simulink model "MeUn_DD"  (R2016b)
settings: configuration reference "CodeGenConfigSet" (kept outside this file)
values from neighbouring files (symbols this model uses):
  DTY_CYC_MIN = fi(0,DutyCycle_rate)    [init_MeUn_DD.m]
  ErrorStatus = fi(0,State_uint8)    [init_MeUn_DD.m]
  MeUn_CrntCtlDT1Kd_C = Calibration.Parameter    [init_MeUn_DD.m]
  MeUn_CrntCtlDT1T1_C = Calibration.Parameter    [init_MeUn_DD.m]
  MeUn_nDiffMax_C = Calibration.Parameter    [init_MeUn_DD.m]
  MeUn_resCoil_C = Calibration.Parameter    [init_MeUn_DD.m]
  MeUn_rPwmOutMax_CUR = Calibration.Parameter    [init_MeUn_DD.m]
  MeUn_rPwmOutMax_CURX = Calibration.Parameter    [init_MeUn_DD.m]
  MeUn_rPwmOutMin_C = Calibration.Parameter    [init_MeUn_DD.m]
  MeUn_rSetLin_CUR = Calibration.Parameter    [init_MeUn_DD.m]
  MeUn_rSetLin_CURX = Calibration.Parameter    [init_MeUn_DD.m]
  MeUn_stHSAct_C = Calibration.Parameter    [init_MeUn_DD.m]
  MeUn_stPwrStgActv_C = Calibration.Parameter    [init_MeUn_DD.m]
  MeUn_stPwrStgDia_C = Calibration.Parameter    [init_MeUn_DD.m]
  MeUn_swtBattCor_C = Calibration.Parameter    [init_MeUn_DD.m]
  MeUn_tiPer_CUR = Calibration.Parameter    [init_MeUn_DD.m]
  MeUn_tiPer_CURX = Calibration.Parameter    [init_MeUn_DD.m]
  MeUn_tiPerUBattHi_C = Calibration.Parameter    [init_MeUn_DD.m]
  MeUn_uBattHi_C = Calibration.Parameter    [init_MeUn_DD.m]
  MeUn_uBattLo_C = Calibration.Parameter    [init_MeUn_DD.m]
  SigTst_rMeUnDuty_C = Calibration.Parameter    [init_MeUn_DD.m]
  SigTst_swtMeUnDuty_C = Calibration.Parameter    [init_MeUn_DD.m]
undefined symbols (not defined in the file or in its folder): Switch_conv
libraries: simulink x4, CXLib x3
settings Model: Creator=Wollf  LastModifiedBy=liutao
settings ConfigSetRef: SourceLocation=Base Workspace

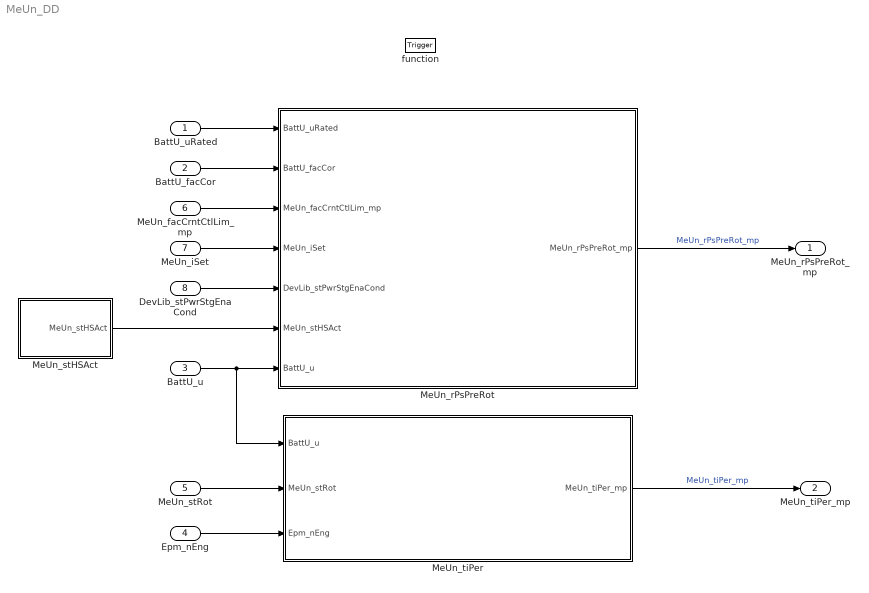
== system MeUn_DD ==
  BattU_uRated : Inport  Tag=mv  Description=Rated battery voltage  OutMin=0  OutMax=50000  OutDataTypeStr=Battery_mv
  BattU_facCor : Inport  Description=Battery correction factor  Port=2  OutMin=-32  OutMax=31.9  OutDataTypeStr=Factor
  BattU_u : Inport  Tag=mv  Description=Battery voltage  Port=3  OutMin=0  OutMax=50000  OutDataTypeStr=Battery_mv
  Epm_nEng : Inport  Tag=rpm  Description=Engine speed  Port=4  OutMin=0  OutMax=6000  OutDataTypeStr=EngSpeed_rpm
  MeUn_stRot : Inport  Description=State of anchor rotation function of metering unit  Port=5  OutMin=0  OutMax=1  OutDataTypeStr=boolean
  MeUn_facCrntCtlLim_mp : Inport  Description=Metering unit current control, I component  Port=6  OutMin=0  OutMax=15  OutDataTypeStr=Pid_Kp_Kd
  MeUn_iSet : Inport  Tag=mA  Description=Setpoint current for the metering unit  Port=7  OutMin=-12000  OutMax=12000  OutDataTypeStr=Current_mA
  DevLib_stPwrStgEnaCond : Inport  Description=Control unit status relevant to power stage deactivation/error diagnosis  Port=8  OutMin=0  OutMax=65535  OutDataTypeStr=State_uint16
  function : TriggerPort  TriggerType=function-call  VariantControl=Variant
  MeUn_rPsPreRot : Subsystem
  MeUn_stHSAct : Subsystem
  MeUn_tiPer : Subsystem
  MeUn_rPsPreRot_mp : Outport  Tag=%  Description=duty cycle of meun current governor before rotation  OutMin=0  OutMax=100  OutDataTypeStr=DutyCycle_rate
  MeUn_tiPer_mp : Outport  Tag=us  Description=Duration of the PWM power stage period  Port=2  OutMin=0  OutMax=6553  OutDataTypeStr=Period_us
  wires:
  MeUn_tiPer/1(MeUn_tiPer_mp) -> MeUn_tiPer_mp/1  "MeUn_tiPer_mp"
  Epm_nEng/1 -> MeUn_tiPer/3(Epm_nEng)
  MeUn_stRot/1 -> MeUn_tiPer/2(MeUn_stRot)
  BattU_uRated/1 -> MeUn_rPsPreRot/1(BattU_uRated)
  BattU_facCor/1 -> MeUn_rPsPreRot/2(BattU_facCor)
  MeUn_facCrntCtlLim_mp/1 -> MeUn_rPsPreRot/3(MeUn_facCrntCtlLim_mp)
  MeUn_iSet/1 -> MeUn_rPsPreRot/4(MeUn_iSet)
  DevLib_stPwrStgEnaCond/1 -> MeUn_rPsPreRot/5(DevLib_stPwrStgEnaCond)
  MeUn_rPsPreRot/1(MeUn_rPsPreRot_mp) -> MeUn_rPsPreRot_mp/1  "MeUn_rPsPreRot_mp"
  BattU_u/1 -> MeUn_tiPer/1(BattU_u), MeUn_rPsPreRot/7(BattU_u)
  MeUn_stHSAct/1(MeUn_stHSAct) -> MeUn_rPsPreRot/6(MeUn_stHSAct)

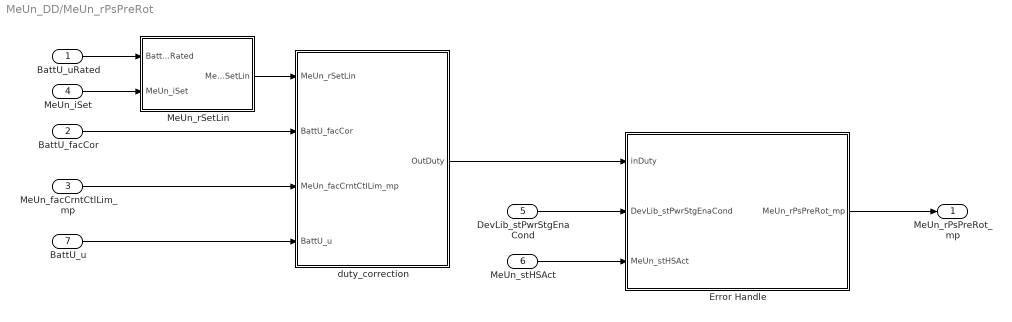
== system MeUn_DD/MeUn_rPsPreRot ==
  BattU_uRated : Inport
  BattU_facCor : Inport  Port=2
  MeUn_facCrntCtlLim_mp : Inport  Port=3
  MeUn_iSet : Inport  Port=4
  DevLib_stPwrStgEnaCond : Inport  Port=5
  MeUn_stHSAct : Inport  Port=6
  BattU_u : Inport  Port=7
  Error Handle : Subsystem  RTWFcnName=error_handle  RTWFileName=error_handle
      settings: RTWSystemCode=Nonreusable function  RTWFcnNameOpts=User specified  RTWFileNameOpts=User specified
  MeUn_rSetLin : Subsystem
  duty_correction : Subsystem
  MeUn_rPsPreRot_mp : Outport
  wires:
  MeUn_rSetLin/1(MeUn_rSetLin) -> duty_correction/1(MeUn_rSetLin)
  MeUn_facCrntCtlLim_mp/1 -> duty_correction/3(MeUn_facCrntCtlLim_mp)
  BattU_facCor/1 -> duty_correction/2(BattU_facCor)
  MeUn_iSet/1 -> MeUn_rSetLin/2(MeUn_iSet)
  BattU_uRated/1 -> MeUn_rSetLin/1(BattU_uRated)
  MeUn_stHSAct/1 -> Error Handle/3(MeUn_stHSAct)
  DevLib_stPwrStgEnaCond/1 -> Error Handle/2(DevLib_stPwrStgEnaCond)
  Error Handle/1(MeUn_rPsPreRot_mp) -> MeUn_rPsPreRot_mp/1
  BattU_u/1 -> duty_correction/4(BattU_u)
  duty_correction/1(OutDuty) -> Error Handle/1(inDuty)

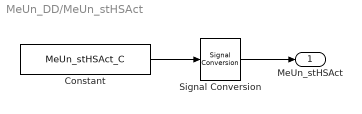
== system MeUn_DD/MeUn_stHSAct ==
  Constant : Constant  Value=MeUn_stHSAct_C
  Signal Conversion : SignalConversion  OverrideOpt=off
  MeUn_stHSAct : Outport
  wires:
  Constant/1 -> Signal Conversion/1
  Signal Conversion/1 -> MeUn_stHSAct/1

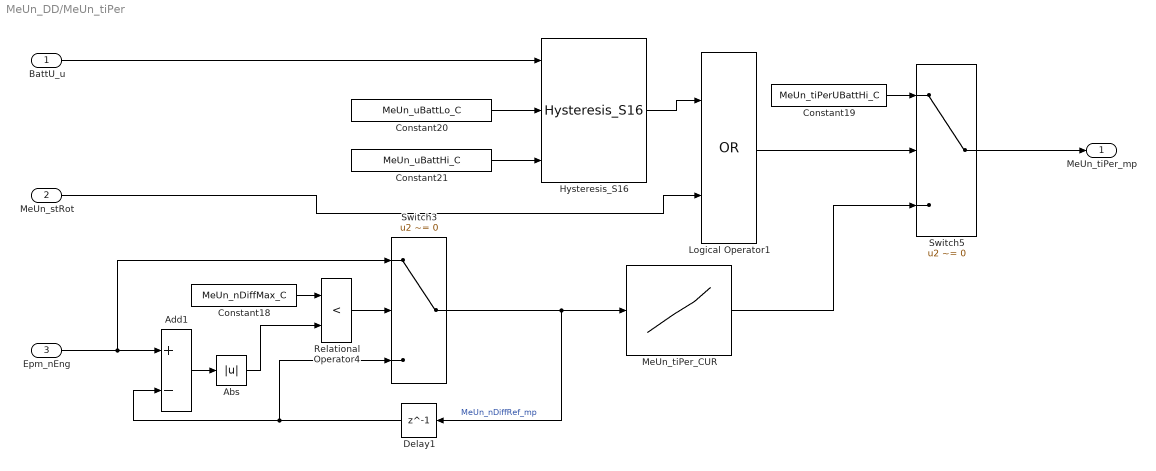
== system MeUn_DD/MeUn_tiPer ==
  BattU_u : Inport
  MeUn_stRot : Inport  Port=2
  Epm_nEng : Inport  Port=3
  Abs : Abs  OutDataTypeStr=Inherit: Inherit via back propagation
  Add1 : Sum  Inputs=+-  OutDataTypeStr=Inherit: Inherit via back propagation  InputSameDT=on
  Constant18 : Constant  Value=MeUn_nDiffMax_C
  Constant19 : Constant  Value=MeUn_tiPerUBattHi_C
  Constant20 : Constant  Value=MeUn_uBattLo_C
  Constant21 : Constant  Value=MeUn_uBattHi_C
  Delay1 : Delay  DelayLength=1  InitialCondition=0
  Hysteresis_S16 : CXLib/Hysteresis_S16
  Logical Operator1 : Logic  Operator=OR  OutDataTypeStr=boolean
  MeUn_tiPer_CUR : Lookup_n-D  NumberOfTableDimensions=1  BreakpointsForDimension1=MeUn_tiPer_CURX  IndexSearchMethod=Linear search  BeginIndexSearchUsingPreviousIndexResult=on  UseOneInputPortForAllInputData=on  Table=MeUn_tiPer_CUR  ExtrapMethod=Clip  UseLastTableValue=on  InternalRulePriority=Speed  OutDataTypeStr=Inherit: Inherit via back propagation  SaturateOnIntegerOverflow=on
  Relational Operator4 : RelationalOperator  Operator=<  OutDataTypeStr=boolean  RndMeth=Nearest  InputSameDT=on
  Switch3 : Switch  Criteria=u2 ~= 0  InputSameDT=on
  Switch5 : Switch  Criteria=u2 ~= 0  InputSameDT=on
  MeUn_tiPer_mp : Outport
  wires:
  MeUn_stRot/1 -> Logical Operator1/2
  Delay1/1 -> Switch3/3, Add1/2
  Switch5/1 -> MeUn_tiPer_mp/1
  MeUn_tiPer_CUR/1 -> Switch5/3
  Hysteresis_S16/1 -> Logical Operator1/1
  Constant20/1 -> Hysteresis_S16/2
  Constant21/1 -> Hysteresis_S16/3
  Logical Operator1/1 -> Switch5/2
  Constant19/1 -> Switch5/1
  Epm_nEng/1 -> Add1/1, Switch3/1
  Relational Operator4/1 -> Switch3/2
  Abs/1 -> Relational Operator4/2
  Constant18/1 -> Relational Operator4/1
  Add1/1 -> Abs/1
  Switch3/1 -> Delay1/1, MeUn_tiPer_CUR/1  "MeUn_nDiffRef_mp"
  BattU_u/1 -> Hysteresis_S16/1

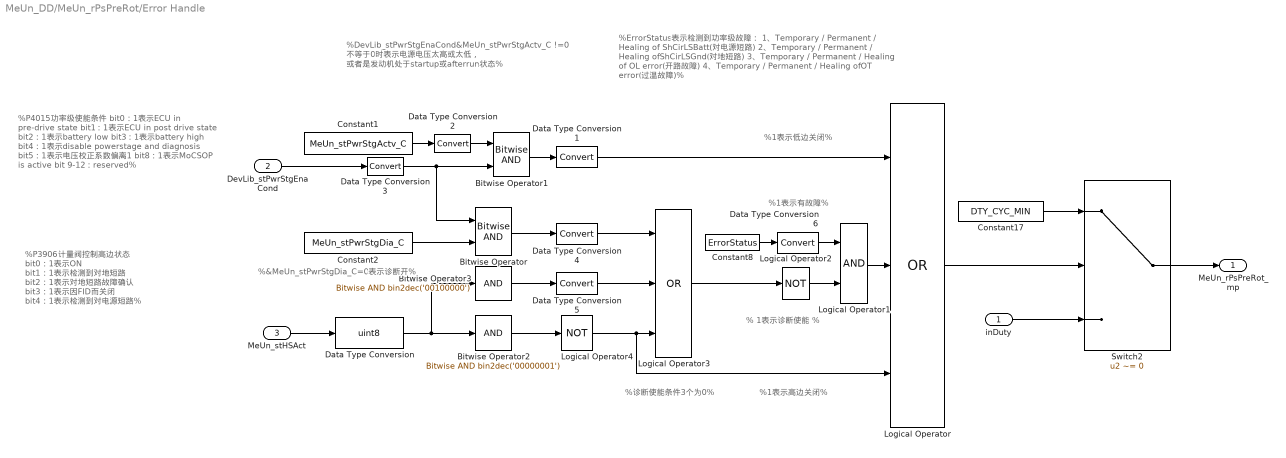
== system MeUn_DD/MeUn_rPsPreRot/Error Handle ==
  note: %1表示高边关闭%
  note: %P4015功率级使能条件
      | bit0：1表示ECU in pre-drive state
      | bit1：1表示ECU in post drive state
      | bit2：1表示battery low
      | bit3：1表示battery high
      | bit4：1表示disable powerstage and diagnosis
      | bit5：1表示电压校正系数偏离1
      | bit8：1表示MoCSOP is active
      | bit 9-12：reserved%
  note: %ErrorStatus表示检测到功率级故障：
      | 1、Temporary / Permanent / Healing of ShCirLSBatt(对电源短路)
      | 2、Temporary / Permanent / Healing ofShCirLSGnd(对地短路)
      | 3、Temporary / Permanent / Healing of OL error(开路故障)
      | 4、Temporary / Permanent / Healing ofOT error(过温故障)%
  note: %P3906计量阀控制高边状态
      | bit0：1表示ON
      | bit1：1表示检测到对地短路
      | bit2：1表示对地短路故障确认
      | bit3：1表示因FID而关闭
      | bit4：1表示检测到对电源短路%
  note: %DevLib_stPwrStgEnaCond&MeUn_stPwrStgActv_C  !=0
      | 不等于0时表示电源电压太高或太低，
      | 或者是发动机处于startup或afterrun状态%
  note: %&MeUn_stPwrStgDia_C=0表示诊断开%
  note: %1表示有故障%
  note: % 1表示诊断使能 %
  note: %诊断使能条件3个为0%
  note: %1表示低边关闭%
  inDuty : Inport
  DevLib_stPwrStgEnaCond : Inport  Port=2
  MeUn_stHSAct : Inport  Port=3
  Bitwise Operator : simulink/Logic and Bit Operations/Bitwise Operator  logicop=AND  UseBitMask=off  NumInputPorts=2  BitMask=bin2dec('00010000')  BitMaskRealWorld=Stored Integer
  Bitwise Operator1 : simulink/Logic and Bit Operations/Bitwise Operator  logicop=AND  UseBitMask=off  NumInputPorts=2  BitMask=bin2dec('00001111')  BitMaskRealWorld=Stored Integer
  Bitwise Operator2 : simulink/Logic and Bit Operations/Bitwise Operator  logicop=AND  UseBitMask=on  BitMask=bin2dec('00000001')  BitMaskRealWorld=Stored Integer
  Bitwise Operator3 : simulink/Logic and Bit Operations/Bitwise Operator  logicop=AND  UseBitMask=on  BitMask=bin2dec('00100000')  BitMaskRealWorld=Stored Integer
  Constant1 : Constant  Value=MeUn_stPwrStgActv_C
  Constant17 : Constant  Value=DTY_CYC_MIN  OutDataTypeStr=Inherit: Inherit via back propagation
  Constant2 : Constant  Value=MeUn_stPwrStgDia_C
  Constant8 : Constant  Value=ErrorStatus  OutDataTypeStr=Inherit: Inherit via back propagation
  Data Type Conversion : DataTypeConversion  OutDataTypeStr=uint8
  Data Type Conversion{1..6} (6 alike) : DataTypeConversion
  Logical Operator : Logic  Operator=OR  Inputs=3  OutDataTypeStr=boolean
  Logical Operator1 : Logic  OutDataTypeStr=boolean
  Logical Operator2 : Logic  Operator=NOT  AllPortsSameDT=off  OutDataTypeStr=boolean
  Logical Operator3 : Logic  Operator=OR  Inputs=3  OutDataTypeStr=boolean
  Logical Operator4 : Logic  Operator=NOT  AllPortsSameDT=off  OutDataTypeStr=boolean
  Switch2 : Switch  Criteria=u2 ~= 0  InputSameDT=on
  MeUn_rPsPreRot_mp : Outport
  wires:
  Data Type Conversion1/1 -> Logical Operator/1
  Data Type Conversion6/1 -> Logical Operator1/1
  Data Type Conversion5/1 -> Logical Operator3/2
  Constant1/1 -> Data Type Conversion2/1
  Data Type Conversion4/1 -> Logical Operator3/1
  Constant2/1 -> Bitwise Operator/2
  Logical Operator4/1 -> Logical Operator3/3, Logical Operator/3
  Bitwise Operator1/1 -> Data Type Conversion1/1
  Bitwise Operator3/1 -> Data Type Conversion5/1
  Bitwise Operator2/1 -> Logical Operator4/1
  MeUn_stHSAct/1 -> Data Type Conversion/1
  DevLib_stPwrStgEnaCond/1 -> Data Type Conversion3/1
  Bitwise Operator/1 -> Data Type Conversion4/1
  Logical Operator3/1 -> Logical Operator2/1
  Logical Operator2/1 -> Logical Operator1/2
  Constant8/1 -> Data Type Conversion6/1
  Logical Operator1/1 -> Logical Operator/2
  Logical Operator/1 -> Switch2/2
  Constant17/1 -> Switch2/1
  Switch2/1 -> MeUn_rPsPreRot_mp/1
  inDuty/1 -> Switch2/3
  Data Type Conversion/1 -> Bitwise Operator2/1, Bitwise Operator3/1
  Data Type Conversion2/1 -> Bitwise Operator1/1
  Data Type Conversion3/1 -> Bitwise Operator1/2, Bitwise Operator/1

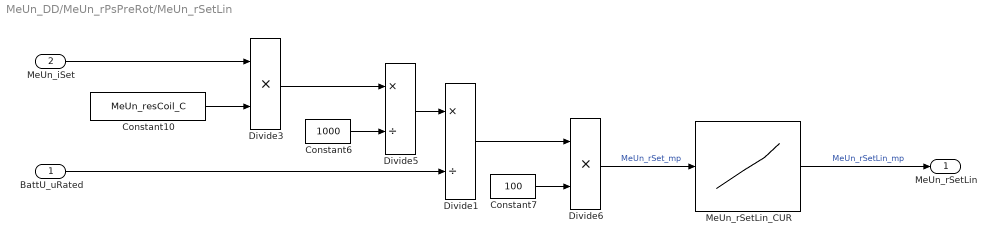
== system MeUn_DD/MeUn_rPsPreRot/MeUn_rSetLin ==
  BattU_uRated : Inport
  MeUn_iSet : Inport  Port=2
  Constant10 : Constant  Value=MeUn_resCoil_C
  Constant6 : Constant  Value=1000  OutDataTypeStr=uint16  SampleTime=-1
  Constant7 : Constant  Value=100  OutDataTypeStr=uint16  SampleTime=-1
  Divide1 : Product  Inputs=*/  OutDataTypeStr=fixdt(0,16,15)  SaturateOnIntegerOverflow=on
  Divide3 : Product  Inputs=**  OutDataTypeStr=fixdt(1,32,0)  SaturateOnIntegerOverflow=on
  Divide5 : Product  Inputs=*/  OutDataTypeStr=Battery_mv  SaturateOnIntegerOverflow=on
  Divide6 : Product  Inputs=**  OutDataTypeStr=DutyCycle_rate  SaturateOnIntegerOverflow=on
  MeUn_rSetLin_CUR : Lookup_n-D  NumberOfTableDimensions=1  BreakpointsForDimension1=MeUn_rSetLin_CURX  IndexSearchMethod=Linear search  BeginIndexSearchUsingPreviousIndexResult=on  UseOneInputPortForAllInputData=on  Table=MeUn_rSetLin_CUR  ExtrapMethod=Clip  UseLastTableValue=on  InternalRulePriority=Speed  OutDataTypeStr=Inherit: Inherit via back propagation  SaturateOnIntegerOverflow=on
  MeUn_rSetLin : Outport
  wires:
  Divide6/1 -> MeUn_rSetLin_CUR/1  "MeUn_rSet_mp"
  MeUn_rSetLin_CUR/1 -> MeUn_rSetLin/1  "MeUn_rSetLin_mp"
  BattU_uRated/1 -> Divide1/2
  Divide5/1 -> Divide1/1
  Constant10/1 -> Divide3/2
  MeUn_iSet/1 -> Divide3/1
  Divide3/1 -> Divide5/1
  Constant6/1 -> Divide5/2
  Divide1/1 -> Divide6/1
  Constant7/1 -> Divide6/2

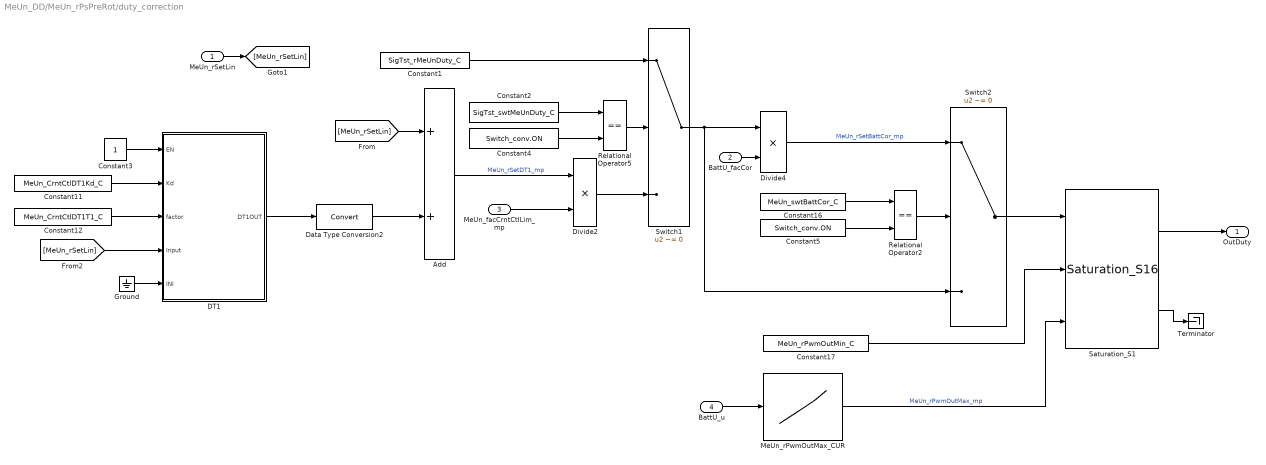
== system MeUn_DD/MeUn_rPsPreRot/duty_correction ==
  MeUn_rSetLin : Inport
  BattU_facCor : Inport  Port=2
  MeUn_facCrntCtlLim_mp : Inport  Port=3
  BattU_u : Inport  Port=4
  Add : Sum  OutDataTypeStr=Inherit: Inherit via back propagation  InputSameDT=on
  Constant1 : Constant  Value=SigTst_rMeUnDuty_C
  Constant11 : Constant  Value=MeUn_CrntCtlDT1Kd_C
  Constant12 : Constant  Value=MeUn_CrntCtlDT1T1_C
  Constant16 : Constant  Value=MeUn_swtBattCor_C
  Constant17 : Constant  Value=MeUn_rPwmOutMin_C
  Constant2 : Constant  Value=SigTst_swtMeUnDuty_C
  Constant3 : Constant  OutDataTypeStr=Inherit: Inherit via back propagation
  Constant4 : Constant  Value=Switch_conv.ON  OutDataTypeStr=Inherit: Inherit via back propagation
  Constant5 : Constant  Value=Switch_conv.ON  OutDataTypeStr=Inherit: Inherit via back propagation
  DT1 : Subsystem
  Data Type Conversion2 : DataTypeConversion  SaturateOnIntegerOverflow=on
  Divide2 : Product  Inputs=**  OutDataTypeStr=DutyCycle_rate
  Divide4 : Product  Inputs=**  OutDataTypeStr=DutyCycle_rate
  Ground : Ground
  MeUn_rPwmOutMax_CUR : Lookup_n-D  NumberOfTableDimensions=1  BreakpointsForDimension1=MeUn_rPwmOutMax_CURX  IndexSearchMethod=Linear search  BeginIndexSearchUsingPreviousIndexResult=on  UseOneInputPortForAllInputData=on  Table=MeUn_rPwmOutMax_CUR  ExtrapMethod=Clip  UseLastTableValue=on  InternalRulePriority=Speed  OutDataTypeStr=Inherit: Inherit via back propagation  SaturateOnIntegerOverflow=on
  Relational Operator2 : RelationalOperator  Operator===  OutDataTypeStr=boolean  RndMeth=Simplest  InputSameDT=on
  Relational Operator5 : RelationalOperator  Operator===  OutDataTypeStr=boolean  RndMeth=Simplest  InputSameDT=on
  Saturation_S1 : CXLib/Saturation_S16
  Switch1 : Switch  Criteria=u2 ~= 0  InputSameDT=on
  Switch2 : Switch  Criteria=u2 ~= 0  InputSameDT=on
  Terminator : Terminator
  OutDuty : Outport
  wires:
  Saturation_S1/1 -> OutDuty/1
  Relational Operator2/1 -> Switch2/2
  Relational Operator5/1 -> Switch1/2
  MeUn_facCrntCtlLim_mp/1 -> Divide2/2
  Constant17/1 -> Saturation_S1/2
  Switch2/1 -> Saturation_S1/1
  Constant16/1 -> Relational Operator2/1
  Divide4/1 -> Switch2/1  "MeUn_rSetBattCor_mp"
  BattU_facCor/1 -> Divide4/2
  Switch1/1 -> Switch2/3, Divide4/1
  Constant1/1 -> Switch1/1
  Divide2/1 -> Switch1/3
  Add/1 -> Divide2/1  "MeUn_rSetDT1_mp"
  Constant2/1 -> Relational Operator5/1
  Constant4/1 -> Relational Operator5/2
  Constant5/1 -> Relational Operator2/2
  DT1/1(DT1OUT) -> Data Type Conversion2/1
  Constant11/1 -> DT1/2(Kd)
  Constant12/1 -> DT1/3(factor)
  MeUn_rPwmOutMax_CUR/1 -> Saturation_S1/3  "MeUn_rPwmOutMax_mp"
  BattU_u/1 -> MeUn_rPwmOutMax_CUR/1
  [MeUn_rSetLin] -> Add/1
  MeUn_rSetLin/1 -> [MeUn_rSetLin]
  Saturation_S1/2 -> Terminator/1
  [MeUn_rSetLin] -> DT1/4(Input)
  Data Type Conversion2/1 -> Add/2
  Constant3/1 -> DT1/1(EN)
  Ground/1 -> DT1/5("INI ")

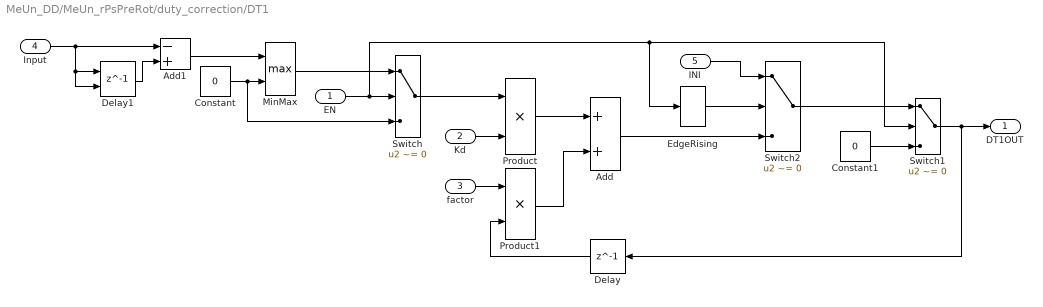
== system MeUn_DD/MeUn_rPsPreRot/duty_correction/DT1 ==
  EN : Inport
  Kd : Inport  Port=2
  factor : Inport  Port=3
  Input : Inport  Port=4
  "INI " : Inport  Port=5
  Add : Sum  OutDataTypeStr=Inherit: Inherit via back propagation  SaturateOnIntegerOverflow=on
  Add1 : Sum  Inputs=-+  OutDataTypeStr=Inherit: Inherit via back propagation  SaturateOnIntegerOverflow=on  InputSameDT=on
  Constant : Constant  Value=0  OutDataTypeStr=Inherit: Inherit via back propagation
  Constant1 : Constant  Value=0  OutDataTypeStr=Inherit: Inherit via back propagation
  Delay : Delay  DelayLength=1  InitialCondition=0
  Delay1 : Delay  DelayLength=1  InitialConditionSource=Input port  InitialCondition=0
      settings: InputPortMap=u0,p4
  EdgeRising : CXLib/EdgeRising
  MinMax : MinMax  Function=max  Inputs=2
  Product : Product  OutDataTypeStr=fixdt(1,32,0.0001,0)  SaturateOnIntegerOverflow=on
  Product1 : Product  OutDataTypeStr=fixdt(1,32,0.0001,0)  SaturateOnIntegerOverflow=on
  Switch : Switch  Criteria=u2 ~= 0  OutDataTypeStr=Inherit: Inherit via back propagation
  Switch1 : Switch  Criteria=u2 ~= 0  InputSameDT=on
  Switch2 : Switch  Criteria=u2 ~= 0  OutDataTypeStr=Inherit: Inherit via back propagation
  DT1OUT : Outport
  wires:
  Kd/1 -> Product/2
  Product/1 -> Add/1
  Constant/1 -> Switch/3, MinMax/2
  Delay/1 -> Product1/2
  Product1/1 -> Add/2
  factor/1 -> Product1/1
  Input/1 -> Add1/1, Delay1/1, Delay1/2
  Delay1/1 -> Add1/2
  Add1/1 -> MinMax/1
  EN/1 -> EdgeRising/1, Switch1/2, Switch/2
  MinMax/1 -> Switch/1
  Switch/1 -> Product/1
  Constant1/1 -> Switch1/3
  Switch1/1 -> Delay/1, DT1OUT/1
  Switch2/1 -> Switch1/1
  Add/1 -> Switch2/3
  EdgeRising/1 -> Switch2/2
  "INI "/1 -> Switch2/1
